simulink model "Test_UKF"  (R2016a)
settings: Solver=FixedStepAuto  StartTime=0.0  StopTime=(stop-start)*dt  FixedStep=0.1  RelTol=1e-3
values from neighbouring files (symbols this model uses):
  alpha = single(0.)    [h.m]    (also in load_sim.m = 0.5; load_test.m = 0.5)
  beta = single(0.)    [h.m]    (also in load_sim.m = 2; load_test.m = 2)
  dt = 0.1    [load_sim.m]    (also in load_test.m)
  ki = 0.00000    (= 0)    [load_sim.m]    (also in load_test.m)
  P0 = diag([0.2 0.2 0.2 0.2 0.2 0.2 0.2])    [load_sim.m]    (also in load_test.m)
  Q = diag([0.100 0.100 0.100 0.01000 0.010 0.010 0.0001].^2)    [load_sim.m]    (also in load_test.m = diag([0.100 0.100 0.100 0.001000 0.0010 0.00010 0.0001].^2))
  R = diag( [0.25000000 0.25000000 0.25000000 0.25000000 0.000004 ] )    [load_sim.m]    (also in load_test.m = diag([0.5000 0.5000 0.8000 0.5000 .002000].^2))
  x0 = zeros(1,7)    [load_sim.m]    (also in load_test.m)
settings Model: Creator=gautier  LastModifiedBy=gautier
settings OptimizationCC: UseDivisionForNetSlopeComputation=on
settings ModelReferenceCC: ModelReferenceNumInstancesAllowed=Single
settings GRTTargetCC: GeneratePreprocessorConditionals=Use local settings

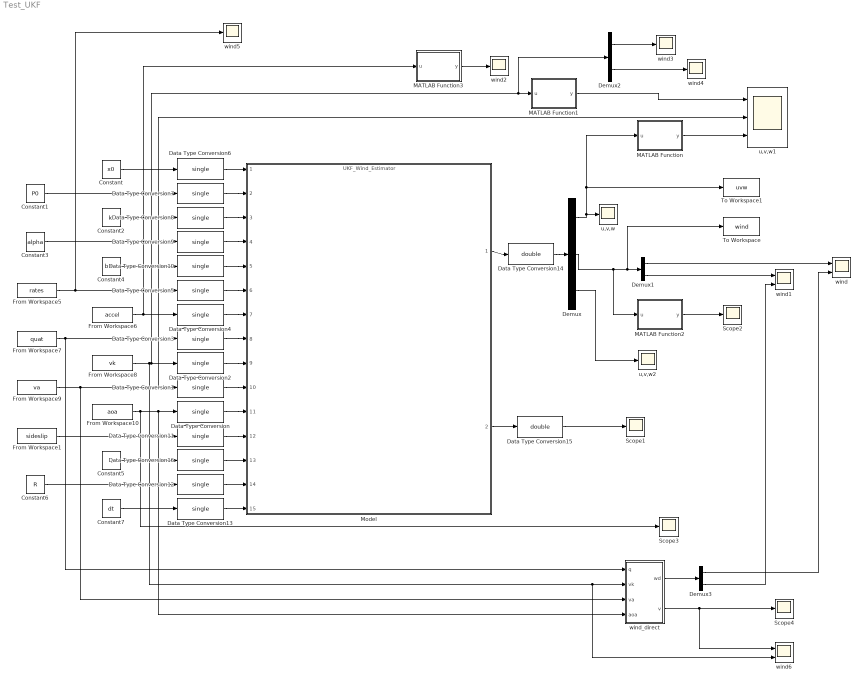
== system Test_UKF ==
  Constant : Constant  Value=x0
  Constant1 : Constant  Value=P0
  Constant2 : Constant  Value=ki
  Constant3 : Constant  Value=alpha
  Constant4 : Constant  Value=beta
  Constant5 : Constant  Value=Q
  Constant6 : Constant  Value=R
  Constant7 : Constant  Value=dt
  Data Type Conversion{,1..13,16} (15 alike) : DataTypeConversion  OutDataTypeStr=single
  Data Type Conversion14 : DataTypeConversion  OutDataTypeStr=double
  Data Type Conversion15 : DataTypeConversion  OutDataTypeStr=double
  Demux : Demux  Outputs=[3 3 1]
  Demux1 : Demux  Outputs=[2 1]
  Demux2 : Demux  Outputs=[2 1]
  Demux3 : Demux  Outputs=[2 1]
  From Workspace1 : FromWorkspace  VariableName=sideslip  SampleTime=dt
  From Workspace10 : FromWorkspace  VariableName=aoa  SampleTime=dt
  From Workspace5 : FromWorkspace  VariableName=rates  SampleTime=dt
  From Workspace6 : FromWorkspace  VariableName=accel  SampleTime=dt
  From Workspace7 : FromWorkspace  VariableName=quat  SampleTime=dt
  From Workspace8 : FromWorkspace  VariableName=vk  SampleTime=dt
  From Workspace9 : FromWorkspace  VariableName=va  SampleTime=dt
  MATLAB Function : MATLAB Function  TreatAsAtomicUnit=on
  MATLAB Function1 : MATLAB Function  TreatAsAtomicUnit=on
  MATLAB Function2 : MATLAB Function  TreatAsAtomicUnit=on
  MATLAB Function3 : MATLAB Function  TreatAsAtomicUnit=on
  Model : ModelReference  ModelNameDialog=UKF_Wind_Estimator.slx  SimulationMode=Normal  ModelReferenceVersion=1.121
  Scope{1..4} (4 alike) : Scope
  To Workspace : ToWorkspace  VariableName=wind  SaveFormat=Timeseries  SampleTime=-1
  To Workspace1 : ToWorkspace  VariableName=uvw  SampleTime=-1
  u,v,w : Scope
  u,v,w1 : Scope  NumInputPorts=3
  u,v,w2 : Scope
  wind : Scope  NumInputPorts=2
  wind1 : Scope  NumInputPorts=2
  wind{2..5} (4 alike) : Scope
  wind6 : Scope  NumInputPorts=2
  wind_direct : MATLAB Function  TreatAsAtomicUnit=on
  wires:
  Constant1/1 -> Data Type Conversion7/1
  Constant2/1 -> Data Type Conversion8/1
  Constant3/1 -> Data Type Conversion9/1
  Constant4/1 -> Data Type Conversion10/1
  From Workspace5/1 -> wind5/1, Data Type Conversion5/1
  From Workspace6/1 -> MATLAB Function3/1(u), Data Type Conversion4/1
  From Workspace7/1 -> wind_direct/1(q), Data Type Conversion3/1
  From Workspace8/1 -> wind6/2, wind_direct/2(vk), Demux2/1, MATLAB Function1/1(u), Data Type Conversion2/1
  From Workspace9/1 -> wind_direct/3(va), u,v,w1/2, Data Type Conversion1/1
  From Workspace10/1 -> Scope3/1, wind_direct/4(aoa), Data Type Conversion/1
  Constant6/1 -> Data Type Conversion12/1
  Constant7/1 -> Data Type Conversion13/1
  Model/1 -> Data Type Conversion14/1
  Model/2 -> Data Type Conversion15/1
  Constant/1 -> Data Type Conversion6/1
  Data Type Conversion/1 -> Model/11
  Data Type Conversion1/1 -> Model/10
  Data Type Conversion2/1 -> Model/9
  Data Type Conversion3/1 -> Model/8
  Data Type Conversion4/1 -> Model/7
  Data Type Conversion5/1 -> Model/6
  Data Type Conversion6/1 -> Model/1
  Data Type Conversion7/1 -> Model/2
  Data Type Conversion8/1 -> Model/3
  Data Type Conversion9/1 -> Model/4
  Data Type Conversion10/1 -> Model/5
  Data Type Conversion11/1 -> Model/12
  Data Type Conversion15/1 -> Scope1/1
  Data Type Conversion14/1 -> Demux/1
  Demux/2 -> To Workspace/1, Demux1/1, MATLAB Function2/1(u)
  Demux/1 -> To Workspace1/1, MATLAB Function/1(u), u,v,w/1
  MATLAB Function1/1(y) -> u,v,w1/1
  MATLAB Function/1(y) -> u,v,w1/3
  MATLAB Function2/1(y) -> Scope2/1
  Demux1/1 -> wind/1
  Demux1/2 -> wind1/1
  MATLAB Function3/1(y) -> wind2/1
  Demux2/1 -> wind3/1
  Demux2/2 -> wind4/1
  wind_direct/1(wd) -> Demux3/1
  Demux3/1 -> wind/2
  Demux3/2 -> wind1/2
  wind_direct/2(v) -> wind6/1, Scope4/1
  Demux/3 -> u,v,w2/1
  Data Type Conversion13/1 -> Model/15
  Data Type Conversion12/1 -> Model/14
  Data Type Conversion16/1 -> Model/13
  Constant5/1 -> Data Type Conversion16/1
  From Workspace1/1 -> Data Type Conversion11/1

== matlab function Test_UKF/MATLAB Function1 ==
  data: u input; y output
function y = fcn(u)
%#codegen

y = norm(u);

== matlab function Test_UKF/MATLAB Function ==
  data: u input; y output
function y = fcn(u)
%#codegen

y = norm(u);

== matlab function Test_UKF/MATLAB Function2 ==
  data: u input; y output
function y = fcn(u)
%#codegen

y = norm(u);

== matlab function Test_UKF/MATLAB Function3 ==
  data: u input; y output
function y = fcn(u)
%#codegen

y = norm(u);

== matlab function Test_UKF/wind_direct ==
  data: q input; wd output; vk input; va input; aoa input; v output
function [wd, v] = fcn(q,vk,va,aoa)
%#codegen
proj=[1 0 tan(aoa)]';
v = (1/0.82)*va*rep2(q,proj);
wd = vk' - v;
